simulink model "UrbanPHIL"  (Simulink 8.1)
settings: Solver=ode1  StartTime=0.0  StopTime=inf  FixedStep=Ts  MaxStep=1e-3  RelTol=1e-3
PostLoadFcn:
  | NREL_Mode=1; BANSHEE_init;
InitFcn:
  | NREL_Mode=1; BANSHEE_init;
values from neighbouring files (symbols this model uses):
  Ts = 100E-6    (= 0.0001)    [BANSHEE_init.m]    (also in Ghost_init.m)
undefined symbols (not defined in the file or in its folder): Hydride, Left, Metal, Nickel, type, V
libraries: powerlib x50, rteventslib x26, rtio_opalrt_op5142ex1 x25, artemis x13, simulink x6, cables_lib x4, relay_housing_lib x3, rtlab x2, utility_service_lib x1, Feeder1_lib x1, Feeder2_lib x1, Feeder3_lib x1
(part 2 of 3)

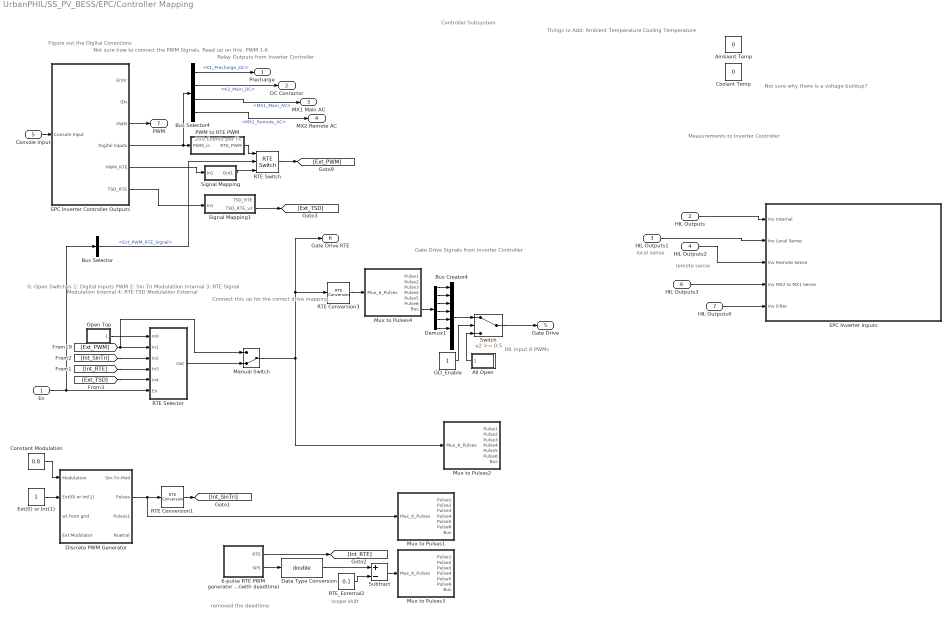
== system UrbanPHIL/SS_PV_BESS/EPC/Controller Mapping ==
  note: Controller Subsystem
  note: Gate Drive Signals from
      | Inverter Controller
  note: Relay Outputs from
      | Inverter Controller
  note: Measurements to
      | Inverter Controller
  note: Not sure why there is a voltage buildup?
  note: Things to Add:
      | Ambient Temperature
      | Cooling Temperature
  note: HIL Input
      | 8 PWMs
  note: local sense
  note: remote sense
  note: Not sure how to connect
      | the PWM Signals.
      | Read up on this.
      | PWM 1-6
  note: Figure out the
      | Digital Conections
  note: removed the deadtime
  note: scope shift
  note: 0; Open Switches
      | 1: Digital Inputs PWM
      | 2: Sin Tri Modulatiion Internal
      | 3: RTE Signal Modulation Internal
      | 4: RTE TSD Modulation External
  note: 200 Events per Ts
  note: Connect this
      | up for the
      | correct drive
      | mapping.
  En : Inport
  HIL Outputs : Inport  Port=2
  HIL Outputs1 : Inport  Port=3
  HIL Outputs2 : Inport  Port=4
  Console Input : Inport  Port=5
  HIL Outputs3 : Inport  Port=6
  HIL Outputs4 : Inport  Port=7
  6-pulse RTE PWM generator (with deadtime) : Subsystem  Tag=RTEcontrol_s38shd7k88  AncestorBlock=|  mask(3-phase RT-Event Discrete PWM Generator){GeneratorMode=3-arm  bridge (6 pulses), Fc=5000, Ts=Ts, mIndex=0.9, Freq=60, Phase=0, Tdead=0}
      | artemis/Tools /Rt-Event 
      | control blocks/6-pulse RTE
      | PWM generator
      | (with deadtime)
      mask prompts: GeneratorMode "Generator Mode"; Fc "Carrier frequency (Hz):"; Ts "Sample time:"; mIndex "Modulation index  (0<m<1) :"; Freq "Frequency of output voltage (Hz)"; Phase "Phase of output voltage (degrees)"; Tdead "Deadtime (s)"
      mask help:
      | This  block generates RT-Event pulses for 3-phase discrete time compensated  carrier-based PWM (Pulse Width Modulation), self-commutated IGBTs,GTOs or FETs bridges in ARTEMIS-RTE.
      |
      | RT-Event pulses are pair of signals that contain the logical value of the switch {on.off} and a timing value used in ARTEMIS-RTE to compensate for in-step switching actions.
      | PSB pulses consist of the logicla part only.
      |
      | Pulses 1,3 and 5 are respectively for the upper switches of the first,second and third arm. Pulses 2,4 and 6 are for the lower switches.
      mask init:
      | set_param(gcb,'LinkStatus','inactive');
      | if Freq==0
      |     Phase=90;
      | end
      |     Internal_Phase=[0 -2*pi/3 2*pi/3];
      |     Signal_PortWidth=3;
      |     Select1_Elements=[1 4 2 5 3 6];
      |     Select1_PortWidth=6;
      |    Select3_Elements=[1 2 3 4 5 6];
      |    Select3_PortWidth=12;
      mask TypeOptions GeneratorMode: 3-arm  bridge (6 pulses)
      mask Display: plot(0,0,100,100,[60,57,57,56,56,53,53,50,50,47,47,41,41,38,38,35,35,32,32,31,31,25,25,24,24,22,22,19,19,16,16,11,11,8,8,5,5,3,3,2,2,0],[20,20,80,80,20,20,80,80,20,20,80,80,20,20,80,80,20,20,80,80,20,20,80,80,20,20,80,80,20,20,80,80,20,20,80,80,20,20,80,80,20,20])
  All Open : Subsystem
  Ambient Temp : Constant  Value=0
  Bus Creator4 : BusCreator  Inputs=8
  Bus Selector : BusSelector  OutputSignals=Ext_PWM_RTE_Signal
  Bus Selector4 : BusSelector  OutputSignals=DIN.DI_CH00-07.K1_Precharge_DC,DIN.DI_CH00-07.K2_Main_DC,DIN.DI_CH00-07.MX1_Main_AC,DIN.DI_CH00-07.MX2_Remote_AC
  Constant Modulation : Constant  Value=0.8
  Coolant Temp : Constant  Value=0
  Data Type Conversion : DataTypeConversion  OutDataTypeStr=double
  Demux1 : Demux  Outputs=6
  Discrete PWM Generator : Subsystem  AncestorBlock=|  DialogController=POWERSYS.PowerSysDialog  mask(Discrete PWM Generator){GeneratorMode=3-arm  bridge (6 pulses), Fc=5000, Ts=Ts, Internal=on, mIndex=0.8, Freq=60, Phase=0}
      | powerlib_extras/Discrete 
      | Control Blocks/Discrete
      | PWM Generator
      mask prompts: GeneratorMode "Generator Mode"; Fc "Carrier frequency (Hz):"; Ts "Sample time:"; Internal "Internal generation of modulating signal(s)"; mIndex "Modulation index  (0<m<1) :"; Freq "Frequency of output voltage (Hz)"; Phase "Phase of output voltage (degrees)"
      mask help:
      | This discrete block generates pulses for carrier-based PWM (Pulse Width Modulation), self-commutated IGBTs,GTOs or FETs bridges.
      |
      | Depending on the number of bridge arms selected in the "Generator Mode" parameter, the block can be used either for single-phase or three-phase PWM control.
      mask init:
      | powericon('psbcallbacks',gcb,'Discrete PWM Generator');
      | if Freq==0
      |     Phase=90;
      | end
      | switch GeneratorMode
      | case 1,
      |     Internal_Phase=0;
      |    Signal_PortWidth=1;
      |    Select1_Elements=[1 2];
      |    Select1_PortWidth=2;
      |    Select3_Elements=[1 2];
      |    Select3_PortWidth=4;
      | case 2,
      |     Internal_Phase=0;
      |     Signal_PortWidth=1;
      |     Select1_Elements=[1 2];
      |     Select1_PortWidth=2;
      |     Select3_Elements=[1 2 3 4];
      |     Select3_PortWidth=4;
      | case 3,
      |     Internal_Phase=[0 -2*pi/3 2*pi/3];
      |     Signal_PortWidth=3;
      |     Select1_Elements=[1 4 2 5 3 6];
      |     Select1_PortWidth=6;
      |    Select3_Elements=[1 2 3 4 5 6];
      |    Select3_PortWidth=12;
      | case 4,
      |     Internal_Phase=[0 -2*pi/3 2*pi/3];
      |     Signal_PortWidth=3;
      |     Select1_Elements=[1 4 2 5 3 6];
      |     Select1_PortWidth=6;
      |    Select3_Elements=[1 2 3 4 5 6 7 8 9 10 11 12];
      |    Select3_PortWidth=12;
      | end
      | power_initmask();
      mask Help:
      | The output pulses are a vector (with values=0 or 1). Depending on the selected "Generator Mode", the output vector contains:
      | For a 1-arm  bridge: Two pulses. Pulse 1 is for the upper switch and pulse 2 is for the lower switch.
      | For a 2-arm  bridge: Four pulses. Pulses 1 and 3 are respectively for the upper switches of the first and second arm. Pulses 2 and 4 are for the lower switches.
      | For a 3-arm  bridge: Six pulses. Pulses 1,3 and 5 are respectively for the upper switches of the first,second and third arm. Pulses 2,4 and 6 are for the lower switches.
      | For double 3-arm bridges: Twelve pulses.The first six pulses (pulses 1 to 6) must be sent to the first 3-arm bridge and the last six (pulses 7 to 12) to the second 3-arm bridge.
      | 
      | By selecting "Internal generation" you can can control the modulation index m, frequency and phase of the output voltage  from the internal parameters (m, Freq and Phase). Otherwise, external signals are used for pulse generation. The width of the input vector must be 1 for single phase bridges ( 1-arm or 2-arm)  and 3 for 3-phase bridges  (single or double bridge).
      mask TypeOptions GeneratorMode: 1-arm  bridge (2 pulses) | 2-arm  bridge (4 pulses) | 3-arm  bridge (6 pulses) | Double 3-arm  bridges (12 pulses)
      mask Callback Internal: %powericon('psbcallbacks',gcb,'Discrete PWM Generator',[]);
      mask Display: disp('')
  EPC Inverter Controller Outputs : Subsystem
  EPC Inverter Inputs : Subsystem
  Ext(0) or Int(1) : Constant
  GD_Enable : Constant
  Manual Switch : ManualSwitch  CurrentSetting=0
  Mux to Pulses1 : Subsystem
  Mux to Pulses2 : Subsystem
  Mux to Pulses3 : Subsystem
  Mux to Pulses4 : Subsystem
  Open Top : Subsystem
  PWM to RTE PWM : Subsystem
  RTE Conversion1 : rteventslib/Signal Attributes/RTE Conversion  inputdatatype=Double  outputdatatype=RTE Boolean  compensation=Enabled  nbMaxEvents=4  sampleTime=Ts
  RTE Conversion3 : rteventslib/Signal Attributes/RTE Conversion  inputdatatype=RTE Boolean  outputdatatype=Double  compensation=Enabled  nbMaxEvents=4  sampleTime=Ts
  RTE Selector : Subsystem
  RTE Switch : rteventslib/Signal Routing/RTE Switch  switchType=u2 = Double; u1 u3 = RTE Boolean  criteria=u2 >= Threshold  threshold=0.5  interpolate=on  nbMaxEvents=4
  RTE_External2 : Constant  Value=0.1
  Signal Mapping : Subsystem
  Signal Mapping1 : Subsystem
  Subtract : Sum  Inputs=+-
  Switch : Switch  Threshold=0.5
  Precharge : Outport
  DC Contactor : Outport  Port=2
  MX1 Main AC : Outport  Port=3
  MX2 Remote AC : Outport  Port=4
  Gate Drive : Outport  Port=5
  Gate Drive RTE : Outport  Port=6
  PWM : Outport  Port=7
  wires:
  Signal Mapping1/2(TSD_RTE_v2) -> [Ext_TSD]
  Demux1/3 -> Bus Creator4/3
  Demux1/5 -> Bus Creator4/5
  GD_Enable/1 -> Switch/2
  Demux1/1 -> Bus Creator4/1
  Demux1/2 -> Bus Creator4/2
  Bus Creator4/1 -> Switch/1
  All Open/1(Pulses8) -> Switch/3
  Demux1/4 -> Bus Creator4/4
  Demux1/6 -> Bus Creator4/6
  HIL Outputs/1 -> EPC Inverter Inputs/1(Inv Internal)
  Console Input/1 -> EPC Inverter Controller Outputs/1(Console Input)
  Constant Modulation/1 -> Discrete PWM Generator/1(Modulation)
  Ext(0) or Int(1)/1 -> Discrete PWM Generator/2(Ext(0) or Int(1))
  6-pulse RTE PWM generator (with deadtime)/1(RTE) -> [Int_RTE]
  RTE Conversion3/1 -> Mux to Pulses4/1(Mux_6_Pulses)
  Mux to Pulses4/7(Bus) -> Demux1/1
  Switch/1 -> Gate Drive/1
  6-pulse RTE PWM generator (with deadtime)/2(SPS) -> Data Type Conversion/1
  Data Type Conversion/1 -> Subtract/1
  RTE_External2/1 -> Subtract/2
  Subtract/1 -> Mux to Pulses3/1(Mux_6_Pulses)
  Bus Selector4/2 -> DC Contactor/1  "<K2_Main_DC>"
  Bus Selector4/1 -> Precharge/1  "<K1_Precharge_DC>"
  EPC Inverter Controller Outputs/3(PWM) -> PWM/1
  RTE Conversion1/1 -> [Int_SinTri]
  Discrete PWM Generator/2(Pulses) -> RTE Conversion1/1, Mux to Pulses1/1(Mux_6_Pulses)
  [Int_SinTri] -> RTE Selector/3(In2)
  Open Top/1(Pulses6) -> RTE Selector/1(In0)
  [Int_RTE] -> RTE Selector/4(In3)
  En/1 -> RTE Selector/6(En), Bus Selector/1
  [Ext_PWM] -> Manual Switch/1, RTE Selector/2(In1)
  RTE Selector/1(Out) -> Manual Switch/2
  Manual Switch/1 -> Mux to Pulses2/1(Mux_6_Pulses), RTE Conversion3/1, Gate Drive RTE/1
  EPC Inverter Controller Outputs/5(PWM_RTE) -> Signal Mapping/1(In1)
  Signal Mapping/1(Out1) -> RTE Switch/3
  RTE Switch/1 -> [Ext_PWM]
  PWM to RTE PWM/1(RTE_PWM) -> RTE Switch/1
  Bus Selector/1 -> RTE Switch/2  "<Ext_PWM_RTE_Signal>"
  EPC Inverter Controller Outputs/4(Digital Inputs) -> Bus Selector4/1, PWM to RTE PWM/1(PWM_in)
  EPC Inverter Controller Outputs/6(TSD_RTE) -> Signal Mapping1/1(In1)
  [Ext_TSD] -> RTE Selector/5(In4)
  HIL Outputs1/1 -> EPC Inverter Inputs/2(Inv Local Sense)
  HIL Outputs2/1 -> EPC Inverter Inputs/3(Inv Remote Sense)
  Bus Selector4/3 -> MX1 Main AC/1  "<MX1_Main_AC>"
  Bus Selector4/4 -> MX2 Remote AC/1  "<MX2_Remote_AC>"
  HIL Outputs3/1 -> EPC Inverter Inputs/4(Inv MX2 to MX1 Sense)
  HIL Outputs4/1 -> EPC Inverter Inputs/5(Inv Filter)

== system UrbanPHIL/SS_PV_BESS/EPC/Inverter_Batt_RTE ==
  note: What does the maximum number of events mean for RTE?
      | What should this be set to?
  note: 1 e-4
      | 1.1 Vf
      | 10 Events
  note: Now 200 Events
  Gate_Drives_RTE : Inport
  Bus Creator1 : BusCreator  Inputs=7
  DC_Bus : powerlib/Elements/Parallel RLC Branch  LConnTagsString=a  RConnTagsString=__new0  BranchType=RC  Resistance=20e3  Inductance=1e-3  SetiL0=off  InitialCurrent=0  Capacitance=2*(925e-6)  Setx0=on  InitialVoltage=0  Measurements=None
  Inv1 : powerlib/Measurements/Current Measurement  PhasorSimulation=off  OutputType=Complex  PSBequivalent=0
  Inv2 : powerlib/Measurements/Current Measurement  PhasorSimulation=off  OutputType=Complex  PSBequivalent=0
  Inv3 : powerlib/Measurements/Current Measurement  PhasorSimulation=off  OutputType=Complex  PSBequivalent=0
  Inv_DC1 : powerlib/Measurements/Current Measurement  PhasorSimulation=off  OutputType=Complex  PSBequivalent=0
  Inv_DC2 : powerlib/Measurements/Current Measurement  PhasorSimulation=off  OutputType=Complex  PSBequivalent=0
  TSB_hiZ snubber_free (contains 6 real diode) : Subsystem
      mask Display: plot(0,0,100,100,[34,34],[60,90],[34,34],[20,50],[60,50],[60,60],[55,59,50,55],[60,50,50,60],[55,55,34],[50,34,34],[34,55,55],[75,75,60],[29,34],[57,50],[23,23,26,23,23,13],[55,51,55,58,55,55])
  V_DClink_1 : powerlib/Measurements/Voltage Measurement  PhasorSimulation=off  OutputType=Complex  PSBequivalent=0
  V_DClink_2 : powerlib/Measurements/Voltage Measurement  PhasorSimulation=off  OutputType=Complex  PSBequivalent=0
  Inv_1 : PMIOPort  Port=1  Side=Left
  Inv_2 : PMIOPort  Port=2  Side=Left
  Inv_3 : PMIOPort  Port=3  Side=Left
  DC+ : PMIOPort  Port=4  Side=Right
  DC- : PMIOPort  Port=5  Side=Right
  m : Outport
  wires:
  Gate_Drives_RTE/1 -> TSB_hiZ snubber_free (contains 6 real diode)/1(g)
  Inv3/1 -> [Inv_Ph3_W_Iout]
  Inv1/1 -> [Inv_Ph1_U_Iout]
  Inv2/1 -> [Inv_Ph2_V_Iout]
  V_DClink_1/1 -> [Inv_Vdc1]
  V_DClink_2/1 -> [Inv_Vdc2]
  Bus Creator1/1 -> m/1
  [Inv_Ph1_U_Iout] -> Bus Creator1/1  "Inv_1"
  [Inv_Ph2_V_Iout] -> Bus Creator1/2  "Inv_2"
  [Inv_Ph3_W_Iout] -> Bus Creator1/3  "Inv_3"
  [Inv_Idc1] -> Bus Creator1/4  "Inv_Idc1"
  [Inv_Idc2] -> Bus Creator1/5  "Inv_Idc2"
  [Inv_Vdc1] -> Bus Creator1/6  "Inv_Vdc1"
  [Inv_Vdc2] -> Bus Creator1/7  "Inv_Vdc2"
  Inv_DC1/1 -> [Inv_Idc1]
  Inv_DC2/1 -> [Inv_Idc2]
  connections:
  Inv_DC1/RConn1 -- TSB_hiZ snubber_free (contains 6 real diode)/RConn1
  TSB_hiZ snubber_free (contains 6 real diode)/LConn1 -- Inv1/RConn1
  TSB_hiZ snubber_free (contains 6 real diode)/LConn2 -- Inv2/RConn1
  TSB_hiZ snubber_free (contains 6 real diode)/LConn3 -- Inv3/RConn1
  DC_Bus/LConn1 -- Inv_DC2/RConn1 -- V_DClink_2/LConn1 -- Inv_DC1/LConn1 -- V_DClink_1/LConn1
  DC+/RConn1 -- Inv_DC2/LConn1
  Inv_1/RConn1 -- Inv1/LConn1
  Inv_2/RConn1 -- Inv2/LConn1
  Inv_3/RConn1 -- Inv3/LConn1
  DC-/RConn1 -- DC_Bus/RConn1 -- V_DClink_2/LConn2 -- TSB_hiZ snubber_free (contains 6 real diode)/RConn2 -- V_DClink_1/LConn2

== system UrbanPHIL/SS_PV_BESS/EPC/LCL Filter 200kW1 ==
  note: High Resistor:
      | 10e6 ohms
      | Numerical Stability
  note: Create a three wire version that removes the Inv 4 port and 4 nuetral.
      | There is a reistor in parallel with the capacitor for the discharge voltage at shutoff.
  Bleed_R1 : powerlib/Elements/Series RLC Branch  LConnTagsString=__new0  RConnTagsString=__new0  BranchType=R  Resistance=filter_cap_bleed_res  Inductance=1e-3  SetiL0=off  InitialCurrent=0  Capacitance=filter_cap  Setx0=on  InitialVoltage=0  Measurements=None
  Bleed_R2 : powerlib/Elements/Series RLC Branch  LConnTagsString=__new0  RConnTagsString=__new0  BranchType=R  Resistance=filter_cap_bleed_res  Inductance=1e-3  SetiL0=off  InitialCurrent=0  Capacitance=filter_cap  Setx0=on  InitialVoltage=0  Measurements=None
  Bleed_R3 : powerlib/Elements/Series RLC Branch  LConnTagsString=__new0  RConnTagsString=__new0  BranchType=R  Resistance=filter_cap_bleed_res  Inductance=1e-3  SetiL0=off  InitialCurrent=0  Capacitance=filter_cap  Setx0=on  InitialVoltage=0  Measurements=None
  Capacitor_L1 : powerlib/Elements/Series RLC Branch  LConnTagsString=__new0  RConnTagsString=__new0  BranchType=RC  Resistance=filter_cap_res  Inductance=1e-3  SetiL0=off  InitialCurrent=0  Capacitance=filter_cap  Setx0=on  InitialVoltage=0  Measurements=None
  Capacitor_L2 : powerlib/Elements/Series RLC Branch  LConnTagsString=__new0  RConnTagsString=__new0  BranchType=RC  Resistance=filter_cap_res  Inductance=1e-3  SetiL0=off  InitialCurrent=0  Capacitance=filter_cap  Setx0=on  InitialVoltage=0  Measurements=None
  Capacitor_L3 : powerlib/Elements/Series RLC Branch  LConnTagsString=__new0  RConnTagsString=__new0  BranchType=RC  Resistance=filter_cap_res  Inductance=1e-3  SetiL0=off  InitialCurrent=0  Capacitance=filter_cap  Setx0=on  InitialVoltage=0  Measurements=None
  Inductor_Inv1 : powerlib/Elements/Series RLC Branch  LConnTagsString=__new0  RConnTagsString=__new0  BranchType=RL  Resistance=filter_inv_res  Inductance=filter_inv_ind  SetiL0=off  InitialCurrent=0  Capacitance=1e-6  Setx0=off  InitialVoltage=0  Measurements=None
  Inductor_Inv2 : powerlib/Elements/Series RLC Branch  LConnTagsString=__new0  RConnTagsString=__new0  BranchType=RL  Resistance=filter_inv_res  Inductance=filter_inv_ind  SetiL0=off  InitialCurrent=0  Capacitance=1e-6  Setx0=off  InitialVoltage=0  Measurements=None
  Inductor_Inv3 : powerlib/Elements/Series RLC Branch  LConnTagsString=__new0  RConnTagsString=__new0  BranchType=RL  Resistance=filter_inv_res  Inductance=filter_inv_ind  SetiL0=off  InitialCurrent=0  Capacitance=1e-6  Setx0=off  InitialVoltage=0  Measurements=None
  Inductor_Inv4 : powerlib/Elements/Series RLC Branch  LConnTagsString=__new0  RConnTagsString=__new0  BranchType=L  Resistance=1  Inductance=filter_inv_ind  SetiL0=off  InitialCurrent=0  Capacitance=1e-6  Setx0=off  InitialVoltage=0  Measurements=None
  Inductor_L1 : powerlib/Elements/Series RLC Branch  LConnTagsString=__new0  RConnTagsString=__new0  BranchType=RL  Resistance=filter_line_res  Inductance=filter_line_ind  SetiL0=off  InitialCurrent=0  Capacitance=1e-6  Setx0=off  InitialVoltage=0  Measurements=None
  Inductor_L2 : powerlib/Elements/Series RLC Branch  LConnTagsString=__new0  RConnTagsString=__new0  BranchType=RL  Resistance=filter_line_res  Inductance=filter_line_ind  SetiL0=off  InitialCurrent=0  Capacitance=1e-6  Setx0=off  InitialVoltage=0  Measurements=None
  Inductor_L3 : powerlib/Elements/Series RLC Branch  LConnTagsString=__new0  RConnTagsString=__new0  BranchType=RL  Resistance=filter_line_res  Inductance=filter_line_ind  SetiL0=off  InitialCurrent=0  Capacitance=1e-6  Setx0=off  InitialVoltage=0  Measurements=None
  Three-Phase Series RLC Branch : powerlib/Elements/Three-Phase Series RLC Branch  LConnTagsString=A|B|C  RConnTagsString=A|B|C  BranchType=R  Resistance=1e6  Inductance=1e-3  Capacitance=1e-6  Measurements=None
  A : PMIOPort  Port=1  Side=Left
  B : PMIOPort  Port=2  Side=Left
  C : PMIOPort  Port=3  Side=Left
  N : PMIOPort  Port=4  Side=Left
  Inv_1 : PMIOPort  Port=5  Side=Right  mask{filter_line_ind=[], filter_cap=0, filter_inv_ind=0}
      mask prompts: filter_line_ind "Line Filter Inductor (H)"; filter_cap "Filter Capacitor (F)"; filter_inv_ind "Inverter Filter Inductor (H)"
  Inv_2 : PMIOPort  Port=6  Side=Right
  Inv_3 : PMIOPort  Port=7  Side=Right
  Inv_4 : PMIOPort  Port=8  Side=Right
  connections:
  Inductor_L1/RConn1 -- Inductor_Inv1/LConn1 -- Capacitor_L1/LConn1 -- Bleed_R1/LConn1
  Inv_1/RConn1 -- Inductor_Inv1/RConn1
  A/RConn1 -- Inductor_L1/LConn1
  Inductor_L2/RConn1 -- Inductor_Inv2/LConn1 -- Capacitor_L2/LConn1 -- Bleed_R2/LConn1
  Inv_2/RConn1 -- Inductor_Inv2/RConn1
  B/RConn1 -- Inductor_L2/LConn1
  Inductor_L3/RConn1 -- Inductor_Inv3/LConn1 -- Capacitor_L3/LConn1 -- Bleed_R3/LConn1
  Inv_3/RConn1 -- Inductor_Inv3/RConn1
  C/RConn1 -- Inductor_L3/LConn1
  N/RConn1 -- Capacitor_L1/RConn1 -- Bleed_R1/RConn1 -- Capacitor_L2/RConn1 -- Bleed_R2/RConn1 -- Capacitor_L3/RConn1 -- Bleed_R3/RConn1 -- Inductor_Inv4/LConn1
  Inv_4/RConn1 -- Inductor_Inv4/RConn1

== system UrbanPHIL/SC_ctrl/EPC Inverter/16TSDIn/16 TSDOut GR3/Din/Dout ch16-23 ==
  Bus Creator3 : BusCreator  Inputs=8
  times17 : Constant  Value=[0.05 0.15 0.25 0.35]
  times18 : Constant  Value=[0.1 0.2 0.3 0.4]
  times19 : Constant  Value=[0.15 0.25 0.35 0.45]
  times20 : Constant  Value=[0.2 0.3 0.4 0.5]
  times21 : Constant  Value=[0.25 0.35 0.45 0.55]
  times22 : Constant  Value=[0.3 0.4 0.5 0.6]
  times23 : Constant  Value=[0.3 0.4 0.5 0.6]
  times24 : Constant  Value=[0 0.1 0.2 0.3]
  Out1 : Outport
  wires:
  times24/1 -> Bus Creator3/1  "times17"
  times17/1 -> Bus Creator3/2  "times18"
  times18/1 -> Bus Creator3/3  "times19"
  times19/1 -> Bus Creator3/4  "times20"
  times20/1 -> Bus Creator3/5  "times21"
  times21/1 -> Bus Creator3/6  "times22"
  times22/1 -> Bus Creator3/7  "times23"
  times23/1 -> Bus Creator3/8  "times24"
  Bus Creator3/1 -> Out1/1

== system UrbanPHIL/SC_ctrl/EPC Inverter/16TSDIn/16 TSDOut GR3/Din/Dout ch24-31 ==
  Bus Creator4 : BusCreator  Inputs=8
  times25 : Constant  Value=[0.05 0.15 0.25 0.35]
  times26 : Constant  Value=[0.1 0.2 0.3 0.4]
  times27 : Constant  Value=[0.15 0.25 0.35 0.45]
  times28 : Constant  Value=[0.2 0.3 0.4 0.5]
  times29 : Constant  Value=[0.25 0.35 0.45 0.55]
  times30 : Constant  Value=[0.3 0.4 0.5 0.6]
  times31 : Constant  Value=[0.3 0.4 0.5 0.6]
  times32 : Constant  Value=[0 0.1 0.2 0.3]
  Out1 : Outport
  wires:
  times32/1 -> Bus Creator4/1  "times25"
  times25/1 -> Bus Creator4/2  "times26"
  times26/1 -> Bus Creator4/3  "times27"
  times27/1 -> Bus Creator4/4  "times28"
  times28/1 -> Bus Creator4/5  "times29"
  times29/1 -> Bus Creator4/6  "times30"
  times30/1 -> Bus Creator4/7  "times31"
  times31/1 -> Bus Creator4/8  "times32"
  Bus Creator4/1 -> Out1/1

== system UrbanPHIL/SC_ctrl/EPC Inverter/16TSDIn/16 TSDOut GR3/Dout state ctrl ==
  Bus Creator : BusCreator  Inputs=2
  Dout_CH16_CH23 : Subsystem
  Dout_CH24_CH31 : Subsystem
  Event State OUT : Outport
  wires:
  Bus Creator/1 -> Event State OUT/1
  Dout_CH16_CH23/1(Dout_CH8_CH15) -> Bus Creator/1  "CH16-23"
  Dout_CH24_CH31/1(Dout_CH8_CH15) -> Bus Creator/2  "CH24-31"

== system UrbanPHIL/SS_PV_BESS/EPC/Controller Mapping/6-pulse RTE PWM generator (with deadtime) ==
  BL4 : Logic  Operator=NOT  Inputs=1
  Constant : Constant  Value=Internal_Phase
  "DeatTime [us] " : Constant  Value=Tdead
  Discrete Triangular-Waveform Generator : Subsystem  mask(Discrete Triangular-Waveform  Generator){Freq=Fc, Vpeak=1, Ts=Ts}
      mask prompts: Freq "Frequency (Hz):"; Vpeak "Peak value:"; Ts "Sample time:"
      mask init:
      | NumberStepsRounded=round(1/Freq/Ts);
      | % Selection of an even number of steps
      | if mod(NumberStepsRounded,2)==0
      |    NumberSteps=NumberStepsRounded;
      | else
      |    NumberSteps=NumberStepsRounded+1;
      | end
      | Freq_used=1/(NumberSteps*Ts);
  Gain : Gain  Gain=2*pi*Freq  SaturateOnIntegerOverflow=on  OutDataTypeStr=Inherit: Same as input  ParamDataTypeStr=Inherit: Same as input
  Gain2 : Gain  Gain=pi/180  SaturateOnIntegerOverflow=on  OutDataTypeStr=Inherit: Same as input  ParamDataTypeStr=Inherit: Same as input
  Mux : Mux  Inputs=2
  Mux2 : Mux  Inputs=2
  Product : Product  SaturateOnIntegerOverflow=on  InputSameDT=on  OutDataTypeStr=Inherit: Same as first input
  RTE Delay1 : rteventslib/Discrete/RTE Delay  IncMode=Enabled  DecMode=Disabled  IC=Low  BufferSize=2  MaxNbEvents=1
  RTE Logical Operator1 : rteventslib/Math Operations/RTE Logical Operator  LogicalOperator=AND  NbrInput=2  NbrMaxEvents=1
  RTE Logical Operator2 : rteventslib/Math Operations/RTE Logical Operator  LogicalOperator=NOR  NbrInput=2  NbrMaxEvents=1
  RTE Relational  Operator : rteventslib/Math Operations/RTE Relational Operator  RelationalOperator=<  NumberMaxEvents=1  SampleTime=Ts
  Relational Operator : RelationalOperator  InputSameDT=on
  Select1A : Selector  InputPortWidth=6  IndexOptions=Index vector (dialog)  Indices=Select1_Elements  OutputSizes=1
  Select1A2 : Selector  InputPortWidth=1  IndexOptions=Index vector (dialog)  Indices=[1 1 1]  OutputSizes=1
  Select1A3 : Selector  InputPortWidth=1  IndexOptions=Index vector (dialog)  Indices=[1 1 1]  OutputSizes=1
  Select1A4 : Selector  InputPortWidth=6  IndexOptions=Index vector (dialog)  Indices=Select1_Elements  OutputSizes=1
  Sum : Sum  Inputs=+++  SaturateOnIntegerOverflow=on  InputSameDT=on  OutDataTypeStr=Inherit: Same as first input
  Terminator1 : Terminator
  Trigonometric Function : Trigonometry
  m3 : Constant  Value=Phase
  m4 : Constant  Value=mIndex
  t : DigitalClock  SampleTime=Ts
  RTE : Outport
  SPS : Outport  Port=2
  wires:
  Select1A4/1 -> RTE/1
  Relational Operator/1 -> Mux/1, BL4/1
  t/1 -> Gain/1
  Gain/1 -> Sum/1
  Gain2/1 -> Sum/2
  m3/1 -> Gain2/1
  Constant/1 -> Sum/3
  m4/1 -> Product/1
  Sum/1 -> Trigonometric Function/1
  Trigonometric Function/1 -> Product/2
  Product/1 -> Relational Operator/1, RTE Relational  Operator/1
  Discrete Triangular-Waveform Generator/2(Freq_used) -> Terminator1/1
  BL4/1 -> Mux/2
  Mux/1 -> Select1A/1
  Discrete Triangular-Waveform Generator/1(Triangle) -> Select1A2/1
  Select1A/1 -> SPS/1
  RTE Logical Operator2/1 -> Mux2/2
  RTE Logical Operator1/1 -> Mux2/1
  RTE Delay1/1 -> RTE Logical Operator1/2, RTE Logical Operator2/2
  "DeatTime [us] "/1 -> Select1A3/1
  RTE Relational  Operator/1 -> RTE Logical Operator2/1, RTE Logical Operator1/1, RTE Delay1/1
  Select1A2/1 -> Relational Operator/2, RTE Relational  Operator/2
  Select1A3/1 -> RTE Delay1/2
  Mux2/1 -> Select1A4/1

== system UrbanPHIL/SS_PV_BESS/EPC/Controller Mapping/All Open ==
  note: This block wiill work for an 8 pulse Sim Power Systems
      | switching model where all are zeros is ok. It will not work
      | with an RTE block because of how the power electronics model.
  Bus Creator1 : BusCreator  Inputs=8
  GD1_8 : Constant  Value=0
  Pulses8 : Outport
  wires:
  GD1_8/1 -> Bus Creator1/1, Bus Creator1/2, Bus Creator1/3, Bus Creator1/4, Bus Creator1/5, Bus Creator1/6, Bus Creator1/7, Bus Creator1/8
  Bus Creator1/1 -> Pulses8/1

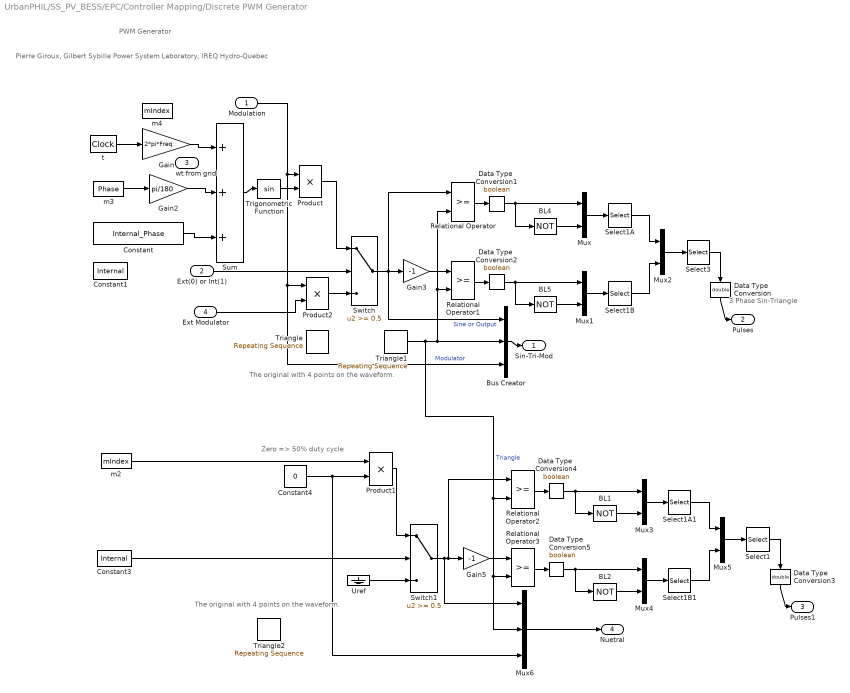
== system UrbanPHIL/SS_PV_BESS/EPC/Controller Mapping/Discrete PWM Generator ==
  note: Pierre Giroux, Gilbert Sybille
      | Power System Laboratory, IREQ
      | Hydro-Quebec
  note: PWM Generator
  note: 3 Phase
      | Sin-Triangle
  note: Zero => 50% duty cycle
  note: The original with 4
      | points on the waveform.
  note: The original with 4
      | points on the waveform.
  Modulation : Inport
  Ext(0) or Int(1) : Inport  Port=2
  wt from grid : Inport  Port=3
  Ext Modulator : Inport  Port=4
  BL{1..2,4..5} (4 alike) : Logic  Operator=NOT  Inputs=1  SampleTime=Ts
  Bus Creator : BusCreator  Inputs=3
  Constant : Constant  Value=Internal_Phase  SampleTime=Ts
  Constant1 : Constant  Value=Internal  SampleTime=Ts
  Constant3 : Constant  Value=Internal  SampleTime=Ts
  Constant4 : Constant  Value=0
  Data Type  Conversion : DataTypeConversion  OutDataTypeStr=double  SampleTime=Ts  SaturateOnIntegerOverflow=on  RndMeth=Zero
  Data Type  Conversion{1..2,4..5} (4 alike) : DataTypeConversion  OutDataTypeStr=boolean  SampleTime=Ts  SaturateOnIntegerOverflow=on  RndMeth=Zero
  Data Type  Conversion3 : DataTypeConversion  OutDataTypeStr=double  SampleTime=Ts  SaturateOnIntegerOverflow=on  RndMeth=Zero
  Gain : Gain  Gain=2*pi*Freq  SaturateOnIntegerOverflow=on  OutDataTypeStr=Inherit: Same as input  ParamDataTypeStr=Inherit: Same as input
  Gain2 : Gain  Gain=pi/180  SaturateOnIntegerOverflow=on  OutDataTypeStr=Inherit: Same as input  ParamDataTypeStr=Inherit: Same as input
  Gain3 : Gain  Gain=-1  SampleTime=Ts  SaturateOnIntegerOverflow=on  OutDataTypeStr=Inherit: Same as input  ParamDataTypeStr=Inherit: Same as input
  Gain5 : Gain  Gain=-1  SampleTime=Ts  SaturateOnIntegerOverflow=on  OutDataTypeStr=Inherit: Same as input  ParamDataTypeStr=Inherit: Same as input
  Mux{,1..5} (6 alike) : Mux  Inputs=2
  Mux6 : Mux  Inputs=3
  Product : Product  SampleTime=Ts  SaturateOnIntegerOverflow=on  InputSameDT=on  OutDataTypeStr=Inherit: Same as first input
  Product1 : Product  SampleTime=Ts  SaturateOnIntegerOverflow=on  InputSameDT=on  OutDataTypeStr=Inherit: Same as first input
  Product2 : Product  SampleTime=Ts  SaturateOnIntegerOverflow=on  InputSameDT=on  OutDataTypeStr=Inherit: Same as first input
  Relational Operator{,1..3} (4 alike) : RelationalOperator  SampleTime=Ts  InputSameDT=on
  Select1 : Selector  InputPortWidth=Select3_PortWidth  IndexOptions=Index vector (dialog)  Indices=Select3_Elements  OutputSizes=1
  Select1A : Selector  InputPortWidth=Select1_PortWidth  IndexOptions=Index vector (dialog)  Indices=Select1_Elements  OutputSizes=1
  Select1A1 : Selector  InputPortWidth=Select1_PortWidth  IndexOptions=Index vector (dialog)  Indices=Select1_Elements  OutputSizes=1
  Select1B : Selector  InputPortWidth=Select1_PortWidth  IndexOptions=Index vector (dialog)  Indices=Select1_Elements  OutputSizes=1
  Select1B1 : Selector  InputPortWidth=Select1_PortWidth  IndexOptions=Index vector (dialog)  Indices=Select1_Elements  OutputSizes=1
  Select3 : Selector  InputPortWidth=Select3_PortWidth  IndexOptions=Index vector (dialog)  Indices=Select3_Elements  OutputSizes=1
  Sum : Sum  Inputs=+++  SampleTime=Ts  SaturateOnIntegerOverflow=on  InputSameDT=on  OutDataTypeStr=Inherit: Same as first input
  Switch : Switch  Threshold=0.5  SampleTime=Ts  SaturateOnIntegerOverflow=on  InputSameDT=on
  Switch1 : Switch  Threshold=0.5  SampleTime=Ts  SaturateOnIntegerOverflow=on  InputSameDT=on
  Triangle : simulink/Sources/Repeating Sequence  rep_seq_t=[0 1/Fc/4 3/Fc/4 1/Fc]  rep_seq_y=[0 -1 1 0]
  Triangle1 : simulink/Sources/Repeating Sequence  rep_seq_t=[0 1/Fc/2 1/Fc]  rep_seq_y=[-1 1 -1]
  Triangle2 : simulink/Sources/Repeating Sequence  rep_seq_t=[0 1/Fc/4 3/Fc/4 1/Fc]  rep_seq_y=[0 -1 1 0]
  Trigonometric Function : Trigonometry  SampleTime=Ts
  Uref : Ground
  m2 : Constant  Value=mIndex  SampleTime=Ts
  m3 : Constant  Value=Phase  SampleTime=Ts
  m4 : Constant  Value=mIndex  SampleTime=Ts
  t : DigitalClock  SampleTime=Ts
  Sin-Tri-Mod : Outport  SampleTime=Ts
  Pulses : Outport  Port=2  SampleTime=Ts
  Pulses1 : Outport  Port=3  SampleTime=Ts
  Nuetral : Outport  Port=4  SampleTime=Ts
  wires:
  Switch/1 -> Relational Operator/1, Gain3/1, Bus Creator/1  "Sine or Output"
  Mux2/1 -> Select3/1
  Select1B/1 -> Mux2/2
  Select1A/1 -> Mux2/1
  Mux1/1 -> Select1B/1
  Mux/1 -> Select1A/1
  BL5/1 -> Mux1/2
  BL4/1 -> Mux/2
  Gain3/1 -> Relational Operator1/1
  Product/1 -> Switch/1
  Trigonometric Function/1 -> Product/2
  Sum/1 -> Trigonometric Function/1
  m3/1 -> Gain2/1
  t/1 -> Gain/1
  Select3/1 -> Data Type  Conversion/1
  Data Type  Conversion/1 -> Pulses/1
  Relational Operator/1 -> Data Type  Conversion1/1
  Data Type  Conversion1/1 -> BL4/1, Mux/1
  Relational Operator1/1 -> Data Type  Conversion2/1
  Data Type  Conversion2/1 -> BL5/1, Mux1/1
  Bus Creator/1 -> Sin-Tri-Mod/1
  Triangle1/1 -> Bus Creator/2, Relational Operator1/2, Relational Operator/2, Relational Operator3/2, Mux6/2, Relational Operator2/2  "Triangle"
  Switch1/1 -> Relational Operator2/1, Gain5/1, Mux6/1
  Mux5/1 -> Select1/1
  Select1B1/1 -> Mux5/2
  Select1A1/1 -> Mux5/1
  Mux4/1 -> Select1B1/1
  Mux3/1 -> Select1A1/1
  BL2/1 -> Mux4/2
  BL1/1 -> Mux3/2
  Gain5/1 -> Relational Operator3/1
  Product1/1 -> Switch1/1
  m2/1 -> Product1/1
  Select1/1 -> Data Type  Conversion3/1
  Data Type  Conversion3/1 -> Pulses1/1
  Relational Operator2/1 -> Data Type  Conversion4/1
  Data Type  Conversion4/1 -> BL1/1, Mux3/1
  Relational Operator3/1 -> Data Type  Conversion5/1
  Data Type  Conversion5/1 -> BL2/1, Mux4/1
  Constant4/1 -> Product1/2, Mux6/3
  Mux6/1 -> Nuetral/1
  Product2/1 -> Switch/3
  Constant3/1 -> Switch1/2
  Uref/1 -> Switch1/3
  Ext(0) or Int(1)/1 -> Switch/2
  Modulation/1 -> Bus Creator/3, Product2/1, Product/1  "Modulator"
  Ext Modulator/1 -> Product2/2
  Constant/1 -> Sum/3
  Gain2/1 -> Sum/2
  Gain/1 -> Sum/1

== system UrbanPHIL/SS_PV_BESS/EPC/Controller Mapping/EPC Inverter Controller Outputs ==
  note: These PWM IN Signals will be used.
      | PWM 1 and 2 are Bot and Top
      | PWM 3 and 4 are Bot and Top
      | PWM 5 and 6 are Bot and Top
  note: When using TSD set the DOUT type config to 0
      | When using PWM set the DOUT type config to 1
  note: It was at 1 for PWM, but it seems that
      | it is better to use the event detector conversion
      | block with TSD instead.
  Console Input : Inport
  Bus Creator1 : BusCreator  Inputs=3
  Bus Creator2 : BusCreator  Inputs=2
  Bus Selector1 : BusSelector  OutputSignals=00-03,04-07  OutputAsBus=on
  Bus Selector2 : BusSelector  OutputSignals=08-11,12-15  OutputAsBus=on
  Bus Selector6 : BusSelector  OutputSignals=16 DOUT GR3,16 TSDOUT GR3,16 PWMOUT GR3
  DIO - Gr4 : Subsystem
  DOUT type config : Subsystem
  GR1 B AIN (CH00-15) : Subsystem
  OpCtrl OP5142EX2 : rtio_opalrt_op5142ex1/OpCtrl OP5142EX1  CtrlName='OP5142EX2 Ctrl'  boardid=2  BitstreamFilename=OP5142_1-EX-0000-2_3_4_54-16AIO_48AO_16DIO_16selDIO_CD-FF-01.bin  numconfig=-1  mode=Slave  externalClock=off  decimRtsi=0  calibIO=off  SampleTime=0  loadinport=-1
  PWM IO - Gr4 : Subsystem
  TSDIO - Gr4 : Subsystem
  Error : Outport
  IDs : Outport  Port=2
  PWM : Outport  Port=3
  Digital Inputs : Outport  Port=4
  PWM_RTE : Outport  Port=5
  TSD_RTE : Outport  Port=6
  wires:
  OpCtrl OP5142EX2/1 -> Error/1
  OpCtrl OP5142EX2/2 -> IDs/1
  PWM IO - Gr4/1(PWMIn) -> Bus Creator1/3, PWM/1  "PWMIN"
  TSDIO - Gr4/1(TSDin) -> Bus Creator1/2  "TSDIN"
  DIO - Gr4/1(DIn) -> Bus Creator1/1  "DIN"
  Bus Creator1/1 -> Digital Inputs/1
  Console Input/1 -> Bus Selector6/1
  Bus Selector6/2 -> TSDIO - Gr4/1(TSDout)  "<16 TSDOUT GR3>"
  Bus Selector6/3 -> PWM IO - Gr4/1(PWMOut)  "<16 PWMOUT GR3>"
  Bus Selector6/1 -> Bus Selector1/1, Bus Selector2/1  "<16 DOUT GR3>"
  Bus Selector1/1 -> Bus Creator2/1  "DI_CH00-07"
  Bus Selector2/1 -> Bus Creator2/2  "DI_CH08-15"
  Bus Creator2/1 -> DIO - Gr4/1(Dout)
  PWM IO - Gr4/2(PWMIn_RTE) -> PWM_RTE/1
  TSDIO - Gr4/2(TSDin_RTE) -> TSD_RTE/1

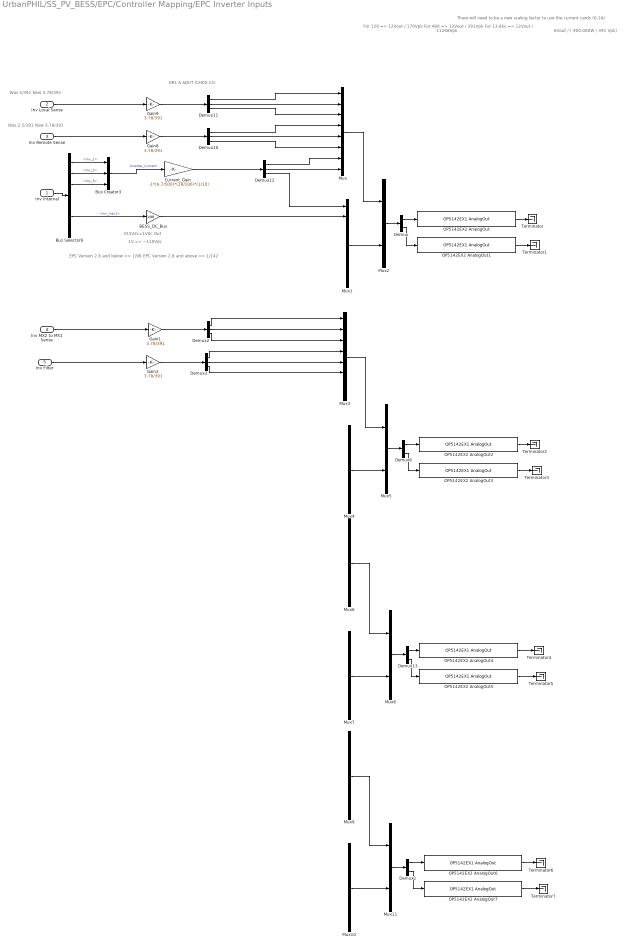
== system UrbanPHIL/SS_PV_BESS/EPC/Controller Mapping/EPC Inverter Inputs ==
  note: 6Vout / ( 900,000W / 391 Vpk)
  note: For 120 => 12Vout / 170Vpk
      | For 480 => 12Vout / 391Vpk
      | For 13.8kv => 12Vout / 11268Vpk
  note: GR1 A AOUT (CH00-15)
  note: There will need to be a
      | new scaling factor to use
      | the current cards (0-1A)
  note: 333Vdc=1Vdc Out
  note: 1V => ~110Vdc
  note: Was 5/391
      | Now 3.78/391
  note: Was 2.5/391
      | Now 3.78/391
  note: EPC Version 2.6 and below => 1/98
      | EPC Version 2.8 and above => 1/142
  Inv Internal : Inport
  Inv Local Sense : Inport  Port=2
  Inv Remote Sense : Inport  Port=3
  Inv MX2 to MX1 Sense : Inport  Port=4
  Inv Filter : Inport  Port=5
  BESS_DC_Bus : Gain  Gain=1/98
  Bus Creator3 : BusCreator  Inputs=3
  Bus Selector6 : BusSelector  OutputSignals=Inv_1,Inv_2,Inv_3,Inv_Idc1,Inv_Idc2,Inv_Vdc1,Inv_Vdc2
  Current_Gain : Gain  Gain=-1*(6.7/500)*(28/106)*(1/10)
  Demux{,1,6,13} (4 alike) : Demux  Outputs=2
  Demux{2..3,10..12} (5 alike) : Demux  Outputs=3
  Gain{1..2,8..9} (4 alike) : Gain  Gain=3.78/391
  Mux{,1,3..4,6..7,9..10} (8 alike) : Mux  Inputs=8
  Mux{2,5,8,11} (4 alike) : Mux  Inputs=2
  OP5142EX2 AnalogOut : rtio_opalrt_op5142ex1/OP5142EX1 AnalogOut  CtrlName='OP5142EX2 Ctrl'  portNb=1  FcnNos=Slot 1 Module A Subsection 1  size=16  maxcount=8  count=8  numchan=8  israngeinput=off  voltagerange=[-16 ... 16]  slot=0  side=0  mismatch=0  slotside=Slot_1_Module_A
      settings: AttributesFormatString=%<CtrlName>
  OP5142EX2 AnalogOut1 : rtio_opalrt_op5142ex1/OP5142EX1 AnalogOut  CtrlName='OP5142EX2 Ctrl'  portNb=2  FcnNos=Slot 1 Module A Subsection 2  size=16  maxcount=8  count=8  numchan=8  israngeinput=off  voltagerange=[-16 ... 16]  slot=0  side=0  mismatch=0  slotside=Slot_1_Module_A
      settings: AttributesFormatString=%<CtrlName>
  OP5142EX2 AnalogOut2 : rtio_opalrt_op5142ex1/OP5142EX1 AnalogOut  CtrlName='OP5142EX2 Ctrl'  portNb=3  FcnNos=Slot 2 Module A Subsection 1  size=16  maxcount=8  count=8  numchan=8  israngeinput=off  voltagerange=[-16 ... 16]  slot=1  side=0  mismatch=0  slotside=Slot_2_Module_A
      settings: AttributesFormatString=%<CtrlName>
  OP5142EX2 AnalogOut3 : rtio_opalrt_op5142ex1/OP5142EX1 AnalogOut  CtrlName='OP5142EX2 Ctrl'  portNb=4  FcnNos=Slot 2 Module A Subsection 2  size=16  maxcount=8  count=8  numchan=8  israngeinput=off  voltagerange=[-16 ... 16]  slot=1  side=0  mismatch=0  slotside=Slot_2_Module_A
      settings: AttributesFormatString=%<CtrlName>
  OP5142EX2 AnalogOut4 : rtio_opalrt_op5142ex1/OP5142EX1 AnalogOut  CtrlName='OP5142EX2 Ctrl'  portNb=5  FcnNos=Slot 2 Module B Subsection 1  size=16  maxcount=8  count=8  numchan=8  israngeinput=off  voltagerange=[-16 ... 16]  slot=1  side=1  mismatch=0  slotside=Slot_2_Module_B
      settings: AttributesFormatString=%<CtrlName>
  OP5142EX2 AnalogOut5 : rtio_opalrt_op5142ex1/OP5142EX1 AnalogOut  CtrlName='OP5142EX2 Ctrl'  portNb=6  FcnNos=Slot 2 Module B Subsection 2  size=16  maxcount=8  count=8  numchan=8  israngeinput=off  voltagerange=[-16 ... 16]  slot=1  side=1  mismatch=0  slotside=Slot_2_Module_B
      settings: AttributesFormatString=%<CtrlName>
  OP5142EX2 AnalogOut6 : rtio_opalrt_op5142ex1/OP5142EX1 AnalogOut  CtrlName='OP5142EX2 Ctrl'  portNb=7  FcnNos=Slot 3 Module A Subsection 1  size=16  maxcount=8  count=8  numchan=8  israngeinput=off  voltagerange=[-16 ... 16]  slot=2  side=0  mismatch=0  slotside=Slot_3_Module_A
      settings: AttributesFormatString=%<CtrlName>
  OP5142EX2 AnalogOut7 : rtio_opalrt_op5142ex1/OP5142EX1 AnalogOut  CtrlName='OP5142EX2 Ctrl'  portNb=8  FcnNos=Slot 3 Module A Subsection 2  size=16  maxcount=8  count=8  numchan=8  israngeinput=off  voltagerange=[-16 ... 16]  slot=2  side=0  mismatch=0  slotside=Slot_3_Module_A
      settings: AttributesFormatString=%<CtrlName>
  Terminator{,1..7} (8 alike) : Terminator
  wires:
  Demux10/3 -> Mux/6
  Demux10/1 -> Mux/4
  Demux10/2 -> Mux/5
  Demux11/3 -> Mux/3
  Demux11/1 -> Mux/1
  Demux11/2 -> Mux/2
  Current_Gain/1 -> Demux12/1
  Mux2/1 -> Demux/1
  Mux1/1 -> Mux2/2
  Mux/1 -> Mux2/1
  Demux/2 -> OP5142EX2 AnalogOut1/1
  Demux/1 -> OP5142EX2 AnalogOut/1
  OP5142EX2 AnalogOut1/1 -> Terminator1/1
  OP5142EX2 AnalogOut/1 -> Terminator/1
  Mux5/1 -> Demux6/1
  Mux4/1 -> Mux5/2
  Mux3/1 -> Mux5/1
  Demux6/2 -> OP5142EX2 AnalogOut3/1
  Demux6/1 -> OP5142EX2 AnalogOut2/1
  OP5142EX2 AnalogOut3/1 -> Terminator3/1
  OP5142EX2 AnalogOut2/1 -> Terminator2/1
  Mux8/1 -> Demux13/1
  Mux7/1 -> Mux8/2
  Mux6/1 -> Mux8/1
  Gain8/1 -> Demux10/1
  Gain9/1 -> Demux11/1
  BESS_DC_Bus/1 -> Mux1/2
  Inv Internal/1 -> Bus Selector6/1
  Inv Local Sense/1 -> Gain9/1
  Inv Remote Sense/1 -> Gain8/1
  Bus Creator3/1 -> Current_Gain/1  "Inverter_Current"
  Demux12/1 -> Mux/7
  Demux12/2 -> Mux/8
  Demux12/3 -> Mux1/1
  Bus Selector6/1 -> Bus Creator3/1  "<Inv_1>"
  Bus Selector6/2 -> Bus Creator3/2  "<Inv_2>"
  Bus Selector6/3 -> Bus Creator3/3  "<Inv_3>"
  Bus Selector6/6 -> BESS_DC_Bus/1  "<Inv_Vdc1>"
  Mux11/1 -> Demux1/1
  Mux10/1 -> Mux11/2
  Mux9/1 -> Mux11/1
  Demux13/1 -> OP5142EX2 AnalogOut4/1
  Demux13/2 -> OP5142EX2 AnalogOut5/1
  OP5142EX2 AnalogOut4/1 -> Terminator4/1
  OP5142EX2 AnalogOut5/1 -> Terminator5/1
  Demux1/1 -> OP5142EX2 AnalogOut6/1
  Demux1/2 -> OP5142EX2 AnalogOut7/1
  OP5142EX2 AnalogOut6/1 -> Terminator6/1
  OP5142EX2 AnalogOut7/1 -> Terminator7/1
  Gain1/1 -> Demux2/1
  Inv MX2 to MX1 Sense/1 -> Gain1/1
  Demux2/1 -> Mux3/1
  Demux2/2 -> Mux3/2
  Demux2/3 -> Mux3/3
  Gain2/1 -> Demux3/1
  Inv Filter/1 -> Gain2/1
  Demux3/1 -> Mux3/4
  Demux3/2 -> Mux3/5
  Demux3/3 -> Mux3/6

== system UrbanPHIL/SS_PV_BESS/EPC/Controller Mapping/Mux to Pulses1 ==
  Mux_6_Pulses : Inport
  Bus Creator24 : BusCreator  Inputs=6
  Bus Selector5 : BusSelector  OutputSignals=Pulse 1,Pukse 2,Pulse 3,Pulse 4,Pulse 5,Pulse 6
  Demux5 : Demux  Outputs=6
  Pulse1 : Outport
  Pulse2 : Outport  Port=2
  Pulse3 : Outport  Port=3
  Pulse4 : Outport  Port=4
  Pulse5 : Outport  Port=5
  Pulse6 : Outport  Port=6
  Bus : Outport  Port=7
  wires:
  Demux5/1 -> Bus Creator24/1  "Pulse 1"
  Demux5/2 -> Bus Creator24/2  "Pukse 2"
  Demux5/3 -> Bus Creator24/3  "Pulse 3"
  Demux5/4 -> Bus Creator24/4  "Pulse 4"
  Demux5/5 -> Bus Creator24/5  "Pulse 5"
  Demux5/6 -> Bus Creator24/6  "Pulse 6"
  Bus Creator24/1 -> Bus Selector5/1, Bus/1
  Mux_6_Pulses/1 -> Demux5/1
  Bus Selector5/1 -> Pulse1/1  "<Pulse 1>"
  Bus Selector5/2 -> Pulse2/1  "<Pukse 2>"
  Bus Selector5/3 -> Pulse3/1  "<Pulse 3>"
  Bus Selector5/4 -> Pulse4/1  "<Pulse 4>"
  Bus Selector5/5 -> Pulse5/1  "<Pulse 5>"
  Bus Selector5/6 -> Pulse6/1  "<Pulse 6>"

== system UrbanPHIL/SS_PV_BESS/EPC/Controller Mapping/Mux to Pulses2 ==
  Mux_6_Pulses : Inport
  Bus Creator24 : BusCreator  Inputs=6
  Bus Selector5 : BusSelector  OutputSignals=Pulse 1,Pukse 2,Pulse 3,Pulse 4,Pulse 5,Pulse 6
  Demux5 : Demux  Outputs=6
  Pulse1 : Outport
  Pulse2 : Outport  Port=2
  Pulse3 : Outport  Port=3
  Pulse4 : Outport  Port=4
  Pulse5 : Outport  Port=5
  Pulse6 : Outport  Port=6
  Bus : Outport  Port=7
  wires:
  Demux5/1 -> Bus Creator24/1  "Pulse 1"
  Demux5/2 -> Bus Creator24/2  "Pukse 2"
  Demux5/3 -> Bus Creator24/3  "Pulse 3"
  Demux5/4 -> Bus Creator24/4  "Pulse 4"
  Demux5/5 -> Bus Creator24/5  "Pulse 5"
  Demux5/6 -> Bus Creator24/6  "Pulse 6"
  Bus Creator24/1 -> Bus Selector5/1, Bus/1
  Mux_6_Pulses/1 -> Demux5/1
  Bus Selector5/1 -> Pulse1/1  "<Pulse 1>"
  Bus Selector5/2 -> Pulse2/1  "<Pukse 2>"
  Bus Selector5/3 -> Pulse3/1  "<Pulse 3>"
  Bus Selector5/4 -> Pulse4/1  "<Pulse 4>"
  Bus Selector5/5 -> Pulse5/1  "<Pulse 5>"
  Bus Selector5/6 -> Pulse6/1  "<Pulse 6>"

== system UrbanPHIL/SS_PV_BESS/EPC/Controller Mapping/Mux to Pulses3 ==
  Mux_6_Pulses : Inport
  Bus Creator24 : BusCreator  Inputs=6
  Bus Selector5 : BusSelector  OutputSignals=Pulse 1,Pukse 2,Pulse 3,Pulse 4,Pulse 5,Pulse 6
  Demux5 : Demux  Outputs=6
  Pulse1 : Outport
  Pulse2 : Outport  Port=2
  Pulse3 : Outport  Port=3
  Pulse4 : Outport  Port=4
  Pulse5 : Outport  Port=5
  Pulse6 : Outport  Port=6
  Bus : Outport  Port=7
  wires:
  Demux5/1 -> Bus Creator24/1  "Pulse 1"
  Demux5/2 -> Bus Creator24/2  "Pukse 2"
  Demux5/3 -> Bus Creator24/3  "Pulse 3"
  Demux5/4 -> Bus Creator24/4  "Pulse 4"
  Demux5/5 -> Bus Creator24/5  "Pulse 5"
  Demux5/6 -> Bus Creator24/6  "Pulse 6"
  Bus Creator24/1 -> Bus Selector5/1, Bus/1
  Mux_6_Pulses/1 -> Demux5/1
  Bus Selector5/1 -> Pulse1/1  "<Pulse 1>"
  Bus Selector5/2 -> Pulse2/1  "<Pukse 2>"
  Bus Selector5/3 -> Pulse3/1  "<Pulse 3>"
  Bus Selector5/4 -> Pulse4/1  "<Pulse 4>"
  Bus Selector5/5 -> Pulse5/1  "<Pulse 5>"
  Bus Selector5/6 -> Pulse6/1  "<Pulse 6>"

== system UrbanPHIL/SS_PV_BESS/EPC/Controller Mapping/Mux to Pulses4 ==
  Mux_6_Pulses : Inport
  Bus Creator24 : BusCreator  Inputs=6
  Bus Selector5 : BusSelector  OutputSignals=Pulse 1,Pukse 2,Pulse 3,Pulse 4,Pulse 5,Pulse 6
  Demux5 : Demux  Outputs=6
  Pulse1 : Outport
  Pulse2 : Outport  Port=2
  Pulse3 : Outport  Port=3
  Pulse4 : Outport  Port=4
  Pulse5 : Outport  Port=5
  Pulse6 : Outport  Port=6
  Bus : Outport  Port=7
  wires:
  Demux5/1 -> Bus Creator24/1  "Pulse 1"
  Demux5/2 -> Bus Creator24/2  "Pukse 2"
  Demux5/3 -> Bus Creator24/3  "Pulse 3"
  Demux5/4 -> Bus Creator24/4  "Pulse 4"
  Demux5/5 -> Bus Creator24/5  "Pulse 5"
  Demux5/6 -> Bus Creator24/6  "Pulse 6"
  Bus Creator24/1 -> Bus Selector5/1, Bus/1
  Mux_6_Pulses/1 -> Demux5/1
  Bus Selector5/1 -> Pulse1/1  "<Pulse 1>"
  Bus Selector5/2 -> Pulse2/1  "<Pukse 2>"
  Bus Selector5/3 -> Pulse3/1  "<Pulse 3>"
  Bus Selector5/4 -> Pulse4/1  "<Pulse 4>"
  Bus Selector5/5 -> Pulse5/1  "<Pulse 5>"
  Bus Selector5/6 -> Pulse6/1  "<Pulse 6>"

== system UrbanPHIL/SS_PV_BESS/EPC/Controller Mapping/Open Top ==
  note: This is for the Gate Drive RTE block. The block does
      | not allow for all the switches to be open at the same time.
  Bus Creator18 : BusCreator  Inputs=6
  GD1_1 : Constant  Value=0
  GD1_2 : Constant
  RTE Conversion2 : rteventslib/Signal Attributes/RTE Conversion  inputdatatype=Double  outputdatatype=RTE Boolean  compensation=Disabled  nbMaxEvents=4  sampleTime=Ts
  Pulses6 : Outport
  wires:
  GD1_1/1 -> Bus Creator18/2, Bus Creator18/6, Bus Creator18/4
  Bus Creator18/1 -> RTE Conversion2/1
  RTE Conversion2/1 -> Pulses6/1
  GD1_2/1 -> Bus Creator18/1, Bus Creator18/3, Bus Creator18/5

== system UrbanPHIL/SS_PV_BESS/EPC/Controller Mapping/PWM to RTE PWM ==
  note: Can one block if mapped
      | or muxed correctly do all
      | of these signals?
      |
      | Check that the correct signal
      | goes to the correct gate.
  PWM_in : Inport
  Bus Creator : BusCreator  Inputs=6
  Bus Selector3 : BusSelector  OutputSignals=PWMIN.PWMI_CH16-23.Freq,PWMIN.PWMI_CH16-23.Duty
  Demux : Demux  Outputs=8
  Demux2 : Demux  Outputs=8
  RTE PWM Bot 1 : rteventslib/Sources/RTE PWM  ShiftedTransition=Enabled  MaxEvents=4  SampleTime=Ts
  RTE PWM Bot 2 : rteventslib/Sources/RTE PWM  ShiftedTransition=Enabled  MaxEvents=4  SampleTime=Ts
  RTE PWM Bot 3 : rteventslib/Sources/RTE PWM  ShiftedTransition=Enabled  MaxEvents=4  SampleTime=Ts
  RTE PWM Top 1 : rteventslib/Sources/RTE PWM  ShiftedTransition=Enabled  MaxEvents=4  SampleTime=Ts
  RTE PWM Top 2 : rteventslib/Sources/RTE PWM  ShiftedTransition=Enabled  MaxEvents=4  SampleTime=Ts
  RTE PWM Top 3 : rteventslib/Sources/RTE PWM  ShiftedTransition=Enabled  MaxEvents=4  SampleTime=Ts
  RTE_PWM : Outport
  wires:
  RTE PWM Bot 3/1 -> Bus Creator/6
  RTE PWM Top 3/1 -> Bus Creator/5
  RTE PWM Bot 2/1 -> Bus Creator/4
  RTE PWM Top 2/1 -> Bus Creator/3
  RTE PWM Bot 1/1 -> Bus Creator/2
  RTE PWM Top 1/1 -> Bus Creator/1
  Demux2/6 -> RTE PWM Bot 3/2
  Demux2/5 -> RTE PWM Top 3/2
  Demux2/4 -> RTE PWM Bot 2/2
  Demux2/3 -> RTE PWM Top 2/2
  Demux2/2 -> RTE PWM Bot 1/2
  Demux/6 -> RTE PWM Bot 3/1
  Demux/5 -> RTE PWM Top 3/1
  Demux/3 -> RTE PWM Top 2/1
  Demux/4 -> RTE PWM Bot 2/1
  Demux/2 -> RTE PWM Bot 1/1
  Demux2/1 -> RTE PWM Top 1/2
  Demux/1 -> RTE PWM Top 1/1
  Bus Selector3/2 -> Demux2/1  "<Duty>"
  Bus Selector3/1 -> Demux/1  "<Freq>"
  Bus Creator/1 -> RTE_PWM/1
  PWM_in/1 -> Bus Selector3/1

== system UrbanPHIL/SS_PV_BESS/EPC/Controller Mapping/RTE Selector ==
  note: MSB
  note: LSB
  In0 : Inport
  In1 : Inport  Port=2
  In2 : Inport  Port=3
  In3 : Inport  Port=4
  In4 : Inport  Port=5
  En : Inport  Port=6
  Bus Selector : BusSelector  OutputSignals=signal1,signal2,signal3,signal4
  RTE Switch{,1..3} (4 alike) : rteventslib/Signal Routing/RTE Switch  switchType=u2 = Double; u1 u3 = RTE Boolean  criteria=u2 >= Threshold  threshold=0.5  interpolate=on  nbMaxEvents=4
  Out : Outport
  wires:
  RTE Switch/1 -> RTE Switch1/1
  RTE Switch1/1 -> RTE Switch2/1
  RTE Switch2/1 -> RTE Switch3/1
  In4/1 -> RTE Switch/1
  In3/1 -> RTE Switch/3
  In2/1 -> RTE Switch1/3
  In1/1 -> RTE Switch2/3
  RTE Switch3/1 -> Out/1
  In0/1 -> RTE Switch3/3
  En/1 -> Bus Selector/1
  Bus Selector/4 -> RTE Switch3/2  "<signal4>"
  Bus Selector/3 -> RTE Switch2/2  "<signal3>"
  Bus Selector/2 -> RTE Switch1/2  "<signal2>"
  Bus Selector/1 -> RTE Switch/2  "<signal1>"

== system UrbanPHIL/SS_PV_BESS/EPC/Controller Mapping/Signal Mapping ==
  In1 : Inport
  Bus Creator : BusCreator  Inputs=6
  Demux : Demux  Outputs=8
  Out1 : Outport
  wires:
  Demux/1 -> Bus Creator/2  "Phase 1 Bot Switch"
  Demux/2 -> Bus Creator/1  "Phase 1 Top Switch"
  Demux/3 -> Bus Creator/4  "Phase 2 Bot Switch"
  Demux/4 -> Bus Creator/3  "Phase 2 Top Switch"
  Demux/5 -> Bus Creator/6  "Phase 3 Bot Switch"
  Demux/6 -> Bus Creator/5  "Phase 3 Top Switch"
  Bus Creator/1 -> Out1/1  "PWM_RTE"
  In1/1 -> Demux/1

== system UrbanPHIL/SS_PV_BESS/EPC/Controller Mapping/Signal Mapping1 ==
  In1 : Inport
  Bus Creator : BusCreator  Inputs=6
  Bus Creator1 : BusCreator  Inputs=6
  Constant : Constant
  Demux : Demux  Outputs=6
  Demux1 : Demux  Outputs=6
  RTE Conversion : rteventslib/Signal Attributes/RTE Conversion  inputdatatype=Double  outputdatatype=RTE Boolean  compensation=Enabled  nbMaxEvents=4  sampleTime=Ts
  RTE Conversion1 : rteventslib/Signal Attributes/RTE Conversion  inputdatatype=RTE Boolean  outputdatatype=Double  compensation=Enabled  nbMaxEvents=4  sampleTime=Ts
  RTE Logical Operator : rteventslib/Math Operations/RTE Logical Operator  LogicalOperator=NOR  NbrInput=6  NbrMaxEvents=4
  RTE Switch : rteventslib/Signal Routing/RTE Switch  switchType=u2 = Double; u1 u3 = RTE Boolean  criteria=u2 >= Threshold  threshold=0.5  interpolate=on  nbMaxEvents=4
  RTE Switch1 : rteventslib/Signal Routing/RTE Switch  switchType=u2 = Double; u1 u3 = RTE Boolean  criteria=u2 >= Threshold  threshold=0.5  interpolate=on  nbMaxEvents=4
  RTE Switch2 : rteventslib/Signal Routing/RTE Switch  switchType=u2 = Double; u1 u3 = RTE Boolean  criteria=u2 >= Threshold  threshold=0.5  interpolate=on  nbMaxEvents=4
  TSD_RTE : Outport
  TSD_RTE_v2 : Outport  Port=2
  wires:
  Bus Creator1/1 -> TSD_RTE_v2/1
  Demux1/6 -> Bus Creator1/6  "Phase 3 Bottom"
  Demux1/5 -> Bus Creator1/5  "Phase 3 Top"
  Demux1/4 -> Bus Creator1/4  "Phase 2 Bottom"
  Demux1/3 -> Bus Creator1/3  "Phase 2 Top"
  Demux1/2 -> Bus Creator1/2  "Phase 1 Bottom"
  Demux1/1 -> Bus Creator1/1  "Phase 1 Top"
  In1/1 -> Demux/1, Demux1/1
  RTE Switch2/1 -> Bus Creator/6
  RTE Switch1/1 -> Bus Creator/4
  RTE Switch/1 -> Bus Creator/2
  Demux/1 -> RTE Logical Operator/1, Bus Creator/1  "Phase 1 Bot Switch"
  Demux/2 -> RTE Logical Operator/2, RTE Switch/3  "Phase 1 Top Switch"
  Demux/3 -> Bus Creator/3, RTE Logical Operator/3  "Phase 2 Bot Switch"
  Demux/4 -> RTE Logical Operator/4, RTE Switch1/3  "Phase 2 Top Switch"
  Demux/5 -> RTE Logical Operator/5, Bus Creator/5  "Phase 3 Bot Switch"
  Demux/6 -> RTE Logical Operator/6, RTE Switch2/3  "Phase 3 Top Switch"
  Bus Creator/1 -> TSD_RTE/1  "TSD_RTE"
  RTE Logical Operator/1 -> RTE Conversion1/1
  Constant/1 -> RTE Conversion/1
  RTE Conversion/1 -> RTE Switch/1, RTE Switch1/1, RTE Switch2/1
  RTE Conversion1/1 -> RTE Switch2/2, RTE Switch/2, RTE Switch1/2
